simulink model "M5_motor_load_gearbox_friction_rated"  (Simulink 10.2)
settings: Solver=ode4  StartTime=0.0  StopTime=3  FixedStep=T_s*0.1  RelTol=1e-3
undefined symbols (not defined in the file): A_v, b_eq, b_v, i_rated, J_eq, k, L, N_opt, omega_v, R, tau_m_rated, theta_0, V_bar
libraries: simulink x1
settings Model: Creator=ioannis  LastModifiedBy=mfocchi
settings DataIOCC: SaveFormat=Dataset  SignalLoggingSaveFormat=Dataset
settings OptimizationCC: LifeSpan=auto
settings DebuggingCC: UnderspecifiedInitializationDetection=Simplified  MergeDetectMultiDrivingBlocksExec=error  FcnCallInpInsideContextMsg=error  SFUnexpectedBacktrackingDiag=error  SFNoUnconditionalDefaultTransitionDiag=error  SFExecutionAtInitializationDiag=warning
settings HardwareCC: ProdBitPerPointer=64  ProdBitPerSizeT=64  ProdBitPerPtrDiffT=64  ProdLargestAtomicFloat=Float  ProdIntDivRoundTo=Zero  ProdEndianess=LittleEndian  ProdWordSize=64  ProdHWDeviceType=Intel->x86-64 (Windows64)
settings ModelReferenceCC: PropagateSignalLabelsOutOfModel=on
settings SFSimCC: SimUseLocalCustomCode=on
settings RTWCC: RTWUseLocalCustomCode=on
settings CodeAppCC: StateflowObjectComments=off
settings GRTTargetCC: TargetLangStandard=C99 (ISO)  CombineOutputUpdateFcns=on  GRTInterface=off
settings ConfigComp: CovMetricSettings=dwe  CovSaveCumulativeToWorkspaceVar=off  CovSaveSingleToWorkspaceVar=off  CovExternalEMLEnable=on

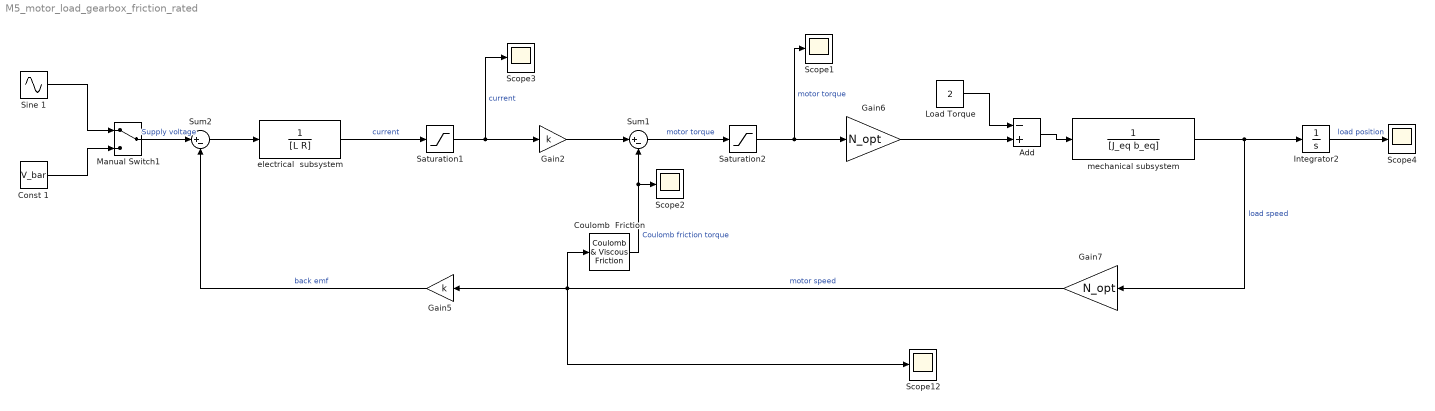
== system M5_motor_load_gearbox_friction_rated ==
  Add : Sum  Inputs=-+
  Const 1 : Constant  Value=V_bar
  Coulomb  Friction : simulink/Discontinuities/Coulomb & Viscous Friction  offset=tau_c  gain=0
  Gain2 : Gain  Gain=k
  Gain5 : Gain  Gain=k
  Gain6 : Gain  Gain=N_opt
  Gain7 : Gain  Gain=N_opt
  Integrator2 : Integrator  InitialCondition=theta_0
  Load Torque : Constant  Value=2
  Manual Switch1 : ManualSwitch
  Saturation1 : Saturate  UpperLimit=i_rated  LowerLimit=-i_rated
  Saturation2 : Saturate  UpperLimit=tau_m_rated  LowerLimit=-tau_m_rated
  Scope{1..4,12} (5 alike) : Scope
  Sine 1 : Sin  Amplitude=A_v  Bias=b_v  Frequency=omega_v  SampleTime=0
  Sum1 : Sum  Inputs=|+-
  Sum2 : Sum  Inputs=|+-
  electrical  subsystem : TransferFcn  Denominator=[L R]
  mechanical subsystem : TransferFcn  Denominator=[J_eq b_eq]
  wires:
  Gain7/1 -> Scope12/1, Coulomb  Friction/1, Gain5/1  "motor speed"
  Manual Switch1/1 -> Sum2/1  "Supply voltage"
  Const 1/1 -> Manual Switch1/2
  mechanical subsystem/1 -> Gain7/1, Integrator2/1  "load speed"
  Gain5/1 -> Sum2/2  "back emf"
  Sine 1/1 -> Manual Switch1/1
  Integrator2/1 -> Scope4/1  "load position"
  Sum2/1 -> electrical  subsystem/1
  Gain2/1 -> Sum1/1
  Coulomb  Friction/1 -> Sum1/2, Scope2/1  "Coulomb friction torque"
  electrical  subsystem/1 -> Saturation1/1  "current"
  Saturation1/1 -> Scope3/1, Gain2/1  "current"
  Sum1/1 -> Saturation2/1  "motor torque"
  Saturation2/1 -> Scope1/1, Gain6/1  "motor torque"
  Load Torque/1 -> Add/1
  Add/1 -> mechanical subsystem/1
  Gain6/1 -> Add/2
